simulink model "modeloSimulink"  (R2021a)
settings: Solver=VariableStepAuto  StartTime=0.0  StopTime=10.0  RelTol=1e-3
values from neighbouring files (symbols this model uses):
  cae = Eq1(1)    [mainVV.m]
  cbe = Eq1(2)    [mainVV.m]
undefined symbols (not defined in the file or in its folder): par
settings Model: Creator=Sergio  LastModifiedBy=Sergio
settings SolverCC: AlgebraicLoopSolver=TrustRegion
settings DataIOCC: ReturnWorkspaceOutputs=off
settings DebuggingCC: SFMachineParentedDataDiag=warning  ArithmeticOperatorsInVariantConditions=warning
settings SFSimCC: SimUseLocalCustomCode=off  CustomCodeUndefinedFunction=UseInterfaceOnly
settings RTWCC: RTWUseLocalCustomCode=off
settings CodeAppCC: StateflowObjectComments=on

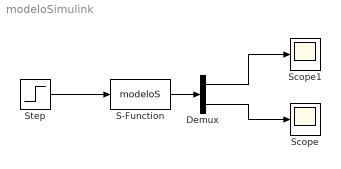
== system modeloSimulink ==
  Demux : Demux  Outputs=2
  S-Function : S-Function  FunctionName=modeloS  Parameters=par,cae,cbe  SFunctionDeploymentMode=off  EnableBusSupport=off
  Scope : Scope
  Scope1 : Scope
  Step : Step  Time=0  Before=4/7  After=4/7+0.01  SampleTime=0
  wires:
  S-Function/1 -> Demux/1
  Step/1 -> S-Function/1
  Demux/1 -> Scope1/1
  Demux/2 -> Scope/1
